simulink model "SensorTemperatura"  (R2013b)
settings: Solver=ode45  StartTime=0.0  StopTime=inf  RelTol=1e-3
undefined symbols (not defined in the file or in its folder): CR, LF, serial
libraries: instrumentlib x2
settings Model: CovHTMLOptions=-sRT=1 -aTS=1 -bRG=1 -bTC=1 -hTR=0 -nFC=0 -scm=1 -bcm=1 -xEv=0  CovModelRefEnable=off  Creator=JorgeAlejandro  LastModifiedBy=JorgeAlejandro

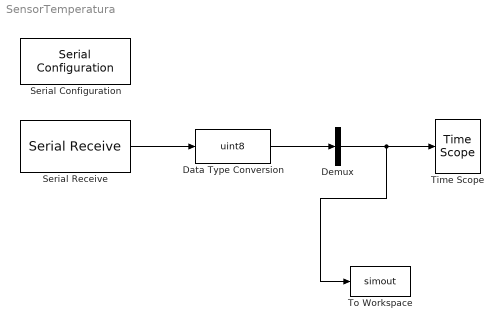
== system SensorTemperatura ==
  Data Type Conversion : DataTypeConversion  OutMin=15  OutMax=15  OutDataTypeStr=uint8
  Demux : Demux  Outputs=1
  Serial Configuration : instrumentlib/Serial Configuration  Priority=-200000  ComPortMenu=COM5  ComPort=COM5  ObjConstructor=serial('COM5');  BaudRate=9600  DataBits=8  Parity=none  StopBits=1  FlowControl=hardware  Timeout=1  ByteOrder=BigEndian
  Serial Receive : instrumentlib/Serial Receive  RequirementInfo={} %GIDa_67db1123_35e5_4315_89cf_a8b8ff1fc4ad  ComPortMenu=COM5  ComPort=COM5  ObjConstructor=serial('COM5');  Header=PS  Terminator=CR/LF ('\r\n')  DataSize=15  DataType=uint8  EnableBlockingMode=on  ActionDataUnavailable=Output last received value  CustomValue=0  SampleTime=0.1
  Time Scope : TimeScope  DefaultConfigurationName=spbscopes.TimeScopeBlockCfg
      settings: CopyFcn=scopeextensions.ScopeBlock.onCoreBlockCopy(gcbh);  DeleteFcn=scopeextensions.ScopeBlock.callback(gcbh, 'onBlockDelete');  PreSaveFcn=scopeextensions.ScopeBlock.callback(gcbh, 'onModelSave');  NameChangeFcn=scopeextensions.ScopeBlock.callback(gcbh, 'onBlockRename');  DestroyFcn=scopeextensions.ScopeBlock.onBlockDestroy(gcbh)  CloseFcn=scopeextensions.ScopeBlock.callback(gcbh, 'onBlockClose');  PreDeleteFcn=scopeextensions.ScopeBlock.callback(gcbh, 'onBlockPreDelete');
  To Workspace : ToWorkspace  VariableName=simout  SampleTime=-1
  wires:
  Demux/1 -> To Workspace/1, Time Scope/1
  Serial Receive/1 -> Data Type Conversion/1
  Data Type Conversion/1 -> Demux/1
